simulink library "PEPS101MSEREF"  (R2014b)
settings: Solver=ode45  StartTime=0.0  StopTime=10.0  RelTol=1e-3
settings Model: Creator=vda2sh  LastModifiedBy=vda2sh

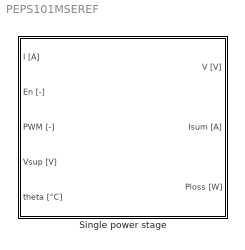
== system PEPS101MSEREF ==
  Single power stage : Subsystem  Tag=PEPS101MSEREF  mask(PEPS101MSEREF){RT20=1e-3, RD20=1e-3, VT20=0, VD20=0.7, IGBT=off, Ieps=1e-3, alphaRT=0, alphaRD=0, alphaVT=0, alphaVD=0}
      mask prompts: RT20 "Transistor on resistance at 20 °C [Ohm]"; RD20 "Diode on resistance at 20 °C [Ohm]"; VT20 "Transistor forward voltage at 20 °C [V]"; VD20 "Diode forward voltage at 20 °C [V]"; IGBT "Enable IGBT"; Ieps "Numerical parameter for diode treatment [A]"; alphaRT "Thermal coefficient of transistor on resistance [1/K]"; alphaRD "Thermal coefficient of diode on resistance [1/K]"; alphaVT "Thermal coefficient of transistor forward voltage [1/K]"; alphaVD "Thermal coefficient of diode forward voltage [1/K]"
      mask help:
      | PEPS101MSEREF - Single power stage
      |
      | This is a model of a power stage with two switches,
      | each switch consisting of a transistor parallel connected to a free-wheel diode.
      settings: AttributesFormatString=<%<Tag>>
      mask Help: eval('show_docs_mseref_powerelectronics(''PEPS101MSEREF'')')
      mask Callback IGBT:
      | % Defining temporary Matlab workspace structure variable `MCBVP__`
      | % `Mask Callback Variable ...` with following fields:
      | % `IGBT`: `0` if Enable IGBT is false, `1` if true
      | % `enables`: `on` if a parameter value can be changed in the mask, `off`
      | % otherwise
      | % `visibilities`: `on` if a parameter may be visible in the mask, `off`
      | % otherwise
      | 
      | % Comparing `IGBT` parameter value with `on`
      | MCBVP__.IGBT = strcmp(get_param(gcb,'IGBT'), 'on');
      | 
      | % Initializing `enables` and `visibilities` fields
      | MCBVP__.enables = {};
      | MCBVP__.visibilities = {};
      | 
      | % Setting `enables` and `visibilities` for `Transistor on resistance at
      | % 20°C`
      | MCBVP__.enables{end + 1} = 'on';
      | MCBVP__.visibilities{end + 1} = 'on';
      | 
      | % Setting `enables` and `visibilities` for `Diode on resistance at 20°C`
      | MCBVP__.enables{end + 1} = 'on';
      | MCBVP__.visibilities{end + 1} = 'on';
      | 
      | % Setting `enables` and `visibilities` for `Transistor forward voltage at 20°C`
      | if MCBVP__.IGBT==true
      |     MCBVP__.enables{end + 1} = 'on';
      |     MCBVP__.visibilities{end + 1} = 'on';
      | else
      |     MCBVP__.enables{end + 1} = 'off';
      |     MCBVP__.visibilities{end + 1} = 'off';
      | end
      | 
      | % Setting `enables` and `visibilities` for `Diode forward voltage at 20°C`
      | MCBVP__.enables{end + 1} = 'on';
      | MCBVP__.visibilities{end + 1} = 'on';
      | 
      | % Setting `enables` and `visibilities` for `IGBT`
      | MCBVP__.enables{end + 1} = 'on';
      | MCBVP__.visibilities{end + 1} = 'on';
      | 
      | % Setting `enables` and `visibilities` for `Numerical parameter for diode treatment`
      | MCBVP__.enables{end + 1} = 'on';
      | MCBVP__.visibilities{end + 1} = 'on';
      | 
      | % Setting `enables` and `visibilities` for `Thermal coefficient of transistor on resistance`
      | MCBVP__.enables{end + 1} = 'on';
      | MCBVP__.visibilities{end + 1} = 'on';
      | 
      | % Setting `enables` and `visibilities` for `Thermal coefficient of diode on resistance`
      | MCBVP__.enables{end + 1} = 'on';
      | MCBVP__.visibilities{end + 1} = 'on';
      | 
      | % Setting `enables` and `visibilities` for `Thermal coefficient of transistor forward voltage`
      | if MCBVP__.IGBT==true
      |     MCBVP__.enables{end + 1} = 'on';
      |     MCBVP__.visibilities{end + 1} = 'on';
      | else
      |     MCBVP__.enables{end + 1} = 'off';
      |     MCBVP__.visibilities{end + 1} = 'off';
      | end
      | 
      | % Setting `enables` and `visibilities` for `Thermal coefficient of diode forward voltage`
      | MCBVP__.enables{end + 1} = 'on';
      | MCBVP__.visibilities{end + 1} = 'on';
      | 
      | % Setting `MaskEnables` and `MaskVisibilities` in current block
      | set_param(gcb, 'MaskEnables', MCBVP__.enables);
      | set_param(gcb, 'MaskVisibilities', MCBVP__.visibilities);
      | 
      | % Clear variable `MCBVP__`
      | clear MCBVP__;
      mask Display:
      | image(imread('PEPS101MSEREF.png'),[0,0, 1,1])
      | text(0.6,0.15, 'MSE')
      | port_label('input',1,'I [A]')
      | port_label('input',2,'En [-]')
      | port_label('input',3,'PWM [-]')
      | port_label('input',4,'Vsup [V]')
      | port_label('input',5,'theta [°C]')
      | port_label('output',1,'V [V]')
      | port_label('output',2,'Isum [A]')
      | port_label('output',3,'Ploss [W]')

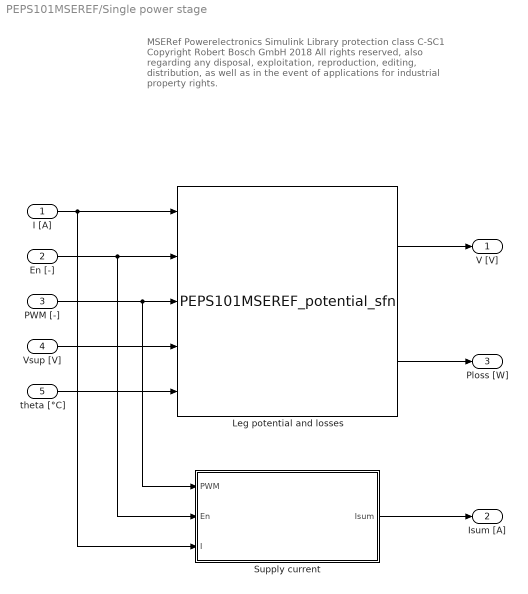
== system PEPS101MSEREF/Single power stage ==
  note: MSERef Powerelectronics Simulink Library
      | protection class C-SC1
      |
      | Copyright Robert Bosch GmbH 2018
      |
      | All rights reserved, also regarding any disposal, exploitation,
      | reproduction, editing, distribution, as well as in the event of
      | applications for industrial property rights.
  I [A] : Inport
  En [-] : Inport  Port=2
  PWM [-] : Inport  Port=3
  Vsup [V] : Inport  Port=4
  theta [°C] : Inport  Port=5
  Leg potential and losses : S-Function  FunctionName=PEPS101MSEREF_potential_sfn  Parameters=RT20, RD20, VT20, VD20, IGBT, Ieps, alphaRT, alphaRD, alphaVT, alphaVD  EnableBusSupport=off  mask(PEPS101MSEREF_potential){RT20=RT20, RD20=RD20, VT20=VT20, VD20=VD20, IGBT=IGBT, Ieps=Ieps, alphaRT=alphaRT, alphaRD=alphaRD, alphaVT=alphaVT, alphaVD=alphaVD}
      mask prompts: RT20 "Transistor on resistance at 20° [Ohm]"; RD20 "Diode on resistance at 20° [Ohm]"; VT20 "Transistor forward voltage at 20° [V]"; VD20 "Diode forward voltage at 20° [V]"; IGBT "Enable IGBT [-]"; Ieps "Numerical parameter for diode treatment [A]"; alphaRT "Thermal coefficient of transistor on resistance [1/K]"; alphaRD "Thermal coefficient of diode on resistance [1/K]"; alphaVT "Thermal coefficient of transistor forward voltage [1/K]"; alphaVD "Thermal coefficient of diode forward voltage [1/K]"
      mask help:
      | This function is used to compute the leg potential and the conduction losses.
      |
      | The `help` button opens the `Single Power Stage` details documentation.
      | With this functionality, a user can open this documentation from the `B6-Bridge` block.
      mask Help: eval('show_docs_mseref_powerelectronics(''PEPS101MSEREF'')')
      mask DialogControl ParameterTabVar0 Prompt: Parameters
      mask Display:
      | text(0.6,0.15, 'MSE')
      | port_label('input',1,'I [A]')
      | port_label('input',2,'En [-]')
      | port_label('input',3,'PWM [-]')
      | port_label('input',4,'Vsup [V]')
      | port_label('input',5,'theta [°C]')
      | port_label('output',1,'V [V]')
      | port_label('output',2,'Ploss [W]')
  Supply current : MATLAB Function  TreatAsAtomicUnit=on
  V [V] : Outport
  Isum [A] : Outport  Port=2
  Ploss [W] : Outport  Port=3
  wires:
  Supply current/1(Isum) -> Isum [A]/1
  Leg potential and losses/2 -> Ploss [W]/1
  Leg potential and losses/1 -> V [V]/1
  theta [°C]/1 -> Leg potential and losses/5
  Vsup [V]/1 -> Leg potential and losses/4
  PWM [-]/1 -> Leg potential and losses/3, Supply current/1(PWM)
  En [-]/1 -> Leg potential and losses/2, Supply current/2(En)
  I [A]/1 -> Leg potential and losses/1, Supply current/3(I)

== matlab function PEPS101MSEREF/Single power stage/Supply current ==
  data: PWM input; Isum output; En input; I input
function Isum = PEPS101MSEREF_supply_current(PWM,En,I)
% This function is used to compute the supply current.
%
%  MSERef Powerelectronics Simulink Library 
%  protection class C-SC1
%
%  Copyright Robert Bosch GmbH 2018
%
%  All rights reserved, also regarding any disposal, exploitation,
%  reproduction, editing, distribution, as well as in the event of
%  applications for industrial property rights.

if ( En >= 0.5 ) % Implementing equation (3)
    Isum = I*PWM;
else % ( En < 0.5 ) % Implementing equation (4)
    Isum = min(I,0);
end
